simulink model "BLDCMotor"  (R2021a)
settings: Solver=VariableStepAuto  StartTime=0.0  StopTime=1  RelTol=1e-3
undefined symbols (not defined in the file): B, backEMFconstant, J, L, R, torqueConstant
settings Model: Creator=ALAKSHENDRA PC  LastModifiedBy=ALAKSHENDRA PC

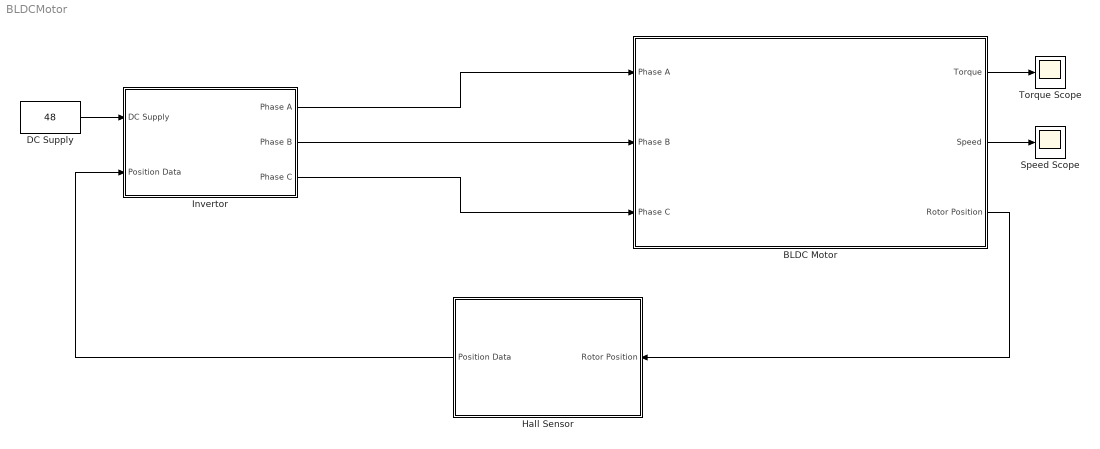
== system BLDCMotor ==
  BLDC Motor : Subsystem
  DC Supply : Constant  Value=48
  Hall Sensor : Subsystem
  Invertor : Subsystem
  Speed Scope : Scope
  Torque Scope : Scope
  wires:
  DC Supply/1 -> Invertor/1(DC Supply)
  Invertor/1(Phase A) -> BLDC Motor/1("Phase A ")
  Invertor/2(Phase B) -> BLDC Motor/2(Phase B)
  Invertor/3(Phase C) -> BLDC Motor/3(Phase C)
  BLDC Motor/3(Rotor Position) -> Hall Sensor/1(Rotor Position)
  Hall Sensor/1(Position Data) -> Invertor/2(Position Data)
  BLDC Motor/1(Torque) -> Torque Scope/1
  BLDC Motor/2(Speed) -> Speed Scope/1

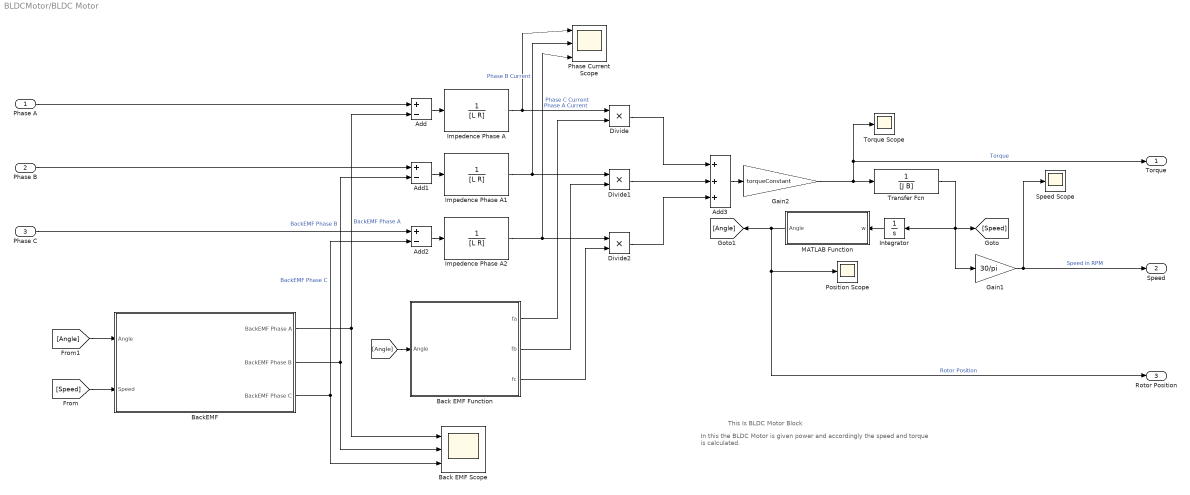
== system BLDCMotor/BLDC Motor ==
  note: This Is BLDC Motor Block
  note: In this the BLDC Motor is given power and accordingly the speed and torque is calculated.
  "Phase A " : Inport
  Phase B : Inport  Port=2
  Phase C : Inport  Port=3
  Add : Sum  Inputs=+-
  Add1 : Sum  Inputs=+-
  Add2 : Sum  Inputs=+-
  Add3 : Sum  Inputs=+++
  Back EMF Function : Subsystem
  Back EMF Scope : Scope  NumInputPorts=3
  BackEMF : Subsystem
  Divide : Product  Inputs=**
  Divide1 : Product  Inputs=**
  Divide2 : Product  Inputs=**
  Gain1 : Gain  Gain=30/pi
  Gain2 : Gain  Gain=torqueConstant
  Impedence Phase A : TransferFcn  Denominator=[L R]
  Impedence Phase A1 : TransferFcn  Denominator=[L R]
  Impedence Phase A2 : TransferFcn  Denominator=[L R]
  Integrator : Integrator
  MATLAB Function : MATLAB Function  TreatAsAtomicUnit=on
  Phase Current Scope : Scope  NumInputPorts=3
  Position Scope : Scope
  Speed Scope : Scope
  Torque Scope : Scope
  Transfer Fcn : TransferFcn  Denominator=[J B]
  Torque : Outport
  Speed : Outport  Port=2
  Rotor Position : Outport  Port=3
  wires:
  Impedence Phase A1/1 -> Divide1/1, Phase Current Scope/2  "Phase B Current"
  [Speed] -> BackEMF/2(Speed)
  BackEMF/2(BackEMF Phase B) -> Back EMF Scope/2, Add1/2  "BackEMF Phase B"
  Add/1 -> Impedence Phase A/1
  Impedence Phase A/1 -> Divide/1, Phase Current Scope/1  "Phase A Current"
  BackEMF/1(BackEMF Phase A) -> Back EMF Scope/1, Add/2  "BackEMF Phase A"
  Back EMF Function/1(fa) -> Divide/2
  BackEMF/3(BackEMF Phase C) -> Back EMF Scope/3, Add2/2  "BackEMF Phase C"
  Back EMF Function/3(fc) -> Divide2/2
  Phase B/1 -> Add1/1
  Add2/1 -> Impedence Phase A2/1
  Integrator/1 -> MATLAB Function/1(w)
  Back EMF Function/2(fb) -> Divide1/2
  Gain2/1 -> Transfer Fcn/1, Torque/1, Torque Scope/1  "Torque"
  Phase C/1 -> Add2/1
  Divide/1 -> Add3/1
  "Phase A "/1 -> Add/1
  MATLAB Function/1(Angle) -> [Angle], Rotor Position/1, Position Scope/1  "Rotor Position"
  Impedence Phase A2/1 -> Divide2/1, Phase Current Scope/3  "Phase C Current"
  Transfer Fcn/1 -> [Speed], Integrator/1, Gain1/1
  Add3/1 -> Gain2/1
  Divide2/1 -> Add3/3
  [Angle] -> Back EMF Function/1(Angle)
  Add1/1 -> Impedence Phase A1/1
  Divide1/1 -> Add3/2
  [Angle] -> BackEMF/1(Angle)
  Gain1/1 -> Speed Scope/1, Speed/1  "Speed in RPM"

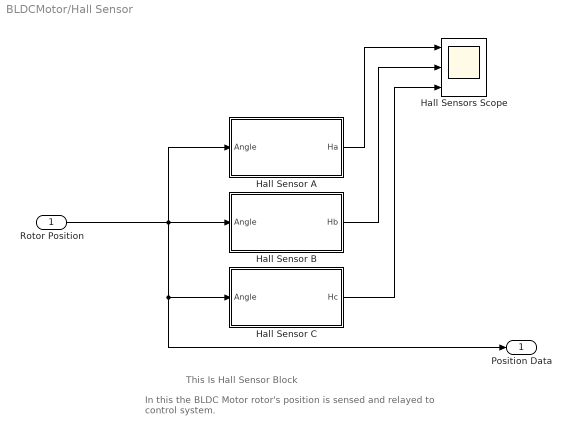
== system BLDCMotor/Hall Sensor ==
  note: This Is Hall Sensor Block
  note: In this the BLDC Motor rotor's position is sensed and relayed to control system.
  Rotor Position : Inport
  Hall Sensor A : MATLAB Function  TreatAsAtomicUnit=on
  Hall Sensor B : MATLAB Function  TreatAsAtomicUnit=on
  Hall Sensor C : MATLAB Function  TreatAsAtomicUnit=on
  Hall Sensors Scope : Scope  NumInputPorts=3
  Position Data : Outport
  wires:
  Hall Sensor B/1(Hb) -> Hall Sensors Scope/2
  Hall Sensor C/1(Hc) -> Hall Sensors Scope/3
  Hall Sensor A/1(Ha) -> Hall Sensors Scope/1
  Rotor Position/1 -> Position Data/1, Hall Sensor C/1(Angle), Hall Sensor A/1(Angle), Hall Sensor B/1(Angle)

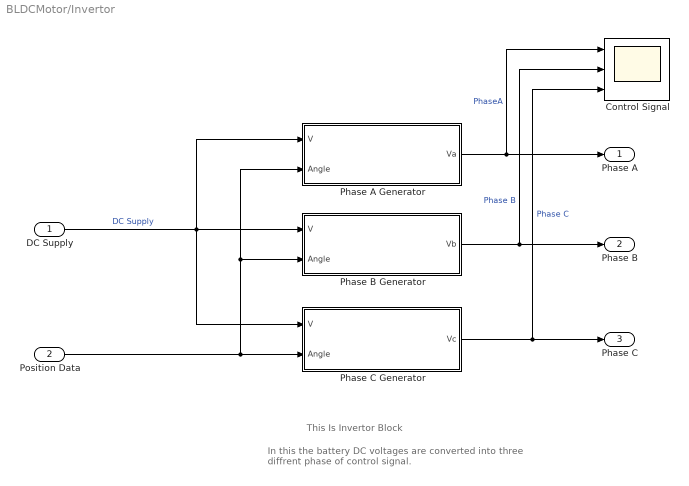
== system BLDCMotor/Invertor ==
  note: In this the battery DC voltages are converted into three diffrent phase of control signal.
  note: This Is Invertor Block
  DC Supply : Inport
  Position Data : Inport  Port=2
  Control Signal : Scope  NumInputPorts=3
  Phase A Generator : MATLAB Function  TreatAsAtomicUnit=on
  Phase B Generator : MATLAB Function  TreatAsAtomicUnit=on
  Phase C Generator : MATLAB Function  TreatAsAtomicUnit=on
  Phase A : Outport
  Phase B : Outport  Port=2
  Phase C : Outport  Port=3
  wires:
  DC Supply/1 -> Phase C Generator/1(V), Phase A Generator/1(V), Phase B Generator/1(V)  "DC Supply"
  Position Data/1 -> Phase A Generator/2(Angle), Phase B Generator/2(Angle), Phase C Generator/2(Angle)
  Phase A Generator/1(Va) -> Control Signal/1, Phase A/1  "PhaseA"
  Phase B Generator/1(Vb) -> Control Signal/2, Phase B/1  "Phase B"
  Phase C Generator/1(Vc) -> Control Signal/3, Phase C/1  "Phase C"

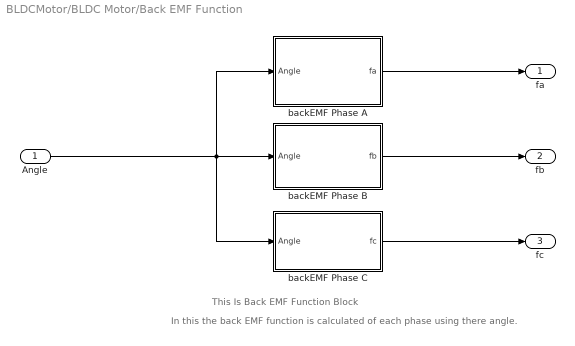
== system BLDCMotor/BLDC Motor/Back EMF Function ==
  note: This Is Back EMF Function Block
  note: In this the back EMF function is calculated of each phase using there angle.
  Angle : Inport
  backEMF Phase A : MATLAB Function  TreatAsAtomicUnit=on
  backEMF Phase B : MATLAB Function  TreatAsAtomicUnit=on
  backEMF Phase C : MATLAB Function  TreatAsAtomicUnit=on
  fa : Outport
  fb : Outport  Port=2
  fc : Outport  Port=3
  wires:
  Angle/1 -> backEMF Phase A/1(Angle), backEMF Phase C/1(Angle), backEMF Phase B/1(Angle)
  backEMF Phase B/1(fb) -> fb/1
  backEMF Phase C/1(fc) -> fc/1
  backEMF Phase A/1(fa) -> fa/1

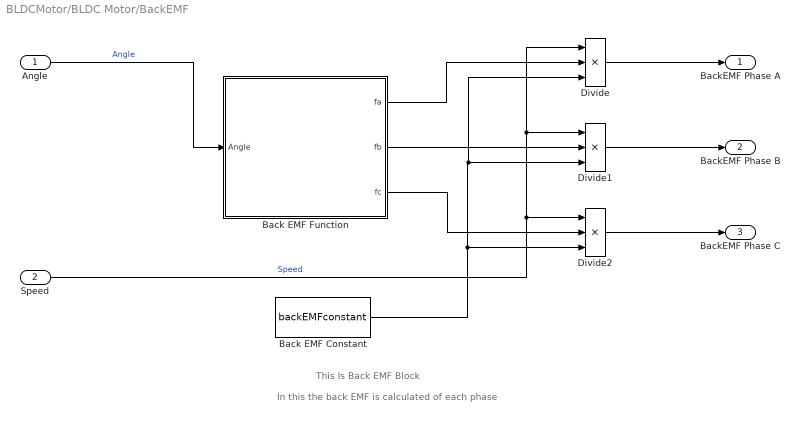
== system BLDCMotor/BLDC Motor/BackEMF ==
  note: This Is Back EMF Block
  note: In this the back EMF is calculated of each phase
  Angle : Inport
  Speed : Inport  Port=2
  Back EMF Constant : Constant  Value=backEMFconstant
  Back EMF Function : Subsystem
  Divide : Product  Inputs=***
  Divide1 : Product  Inputs=***
  Divide2 : Product  Inputs=***
  BackEMF Phase A : Outport
  BackEMF Phase B : Outport  Port=2
  BackEMF Phase C : Outport  Port=3
  wires:
  Back EMF Constant/1 -> Divide/3, Divide1/3, Divide2/3
  Divide1/1 -> BackEMF Phase B/1
  Divide/1 -> BackEMF Phase A/1
  Divide2/1 -> BackEMF Phase C/1
  Speed/1 -> Divide1/1, Divide/1, Divide2/1  "Speed"
  Angle/1 -> Back EMF Function/1(Angle)  "Angle"
  Back EMF Function/1(fa) -> Divide/2
  Back EMF Function/2(fb) -> Divide1/2
  Back EMF Function/3(fc) -> Divide2/2

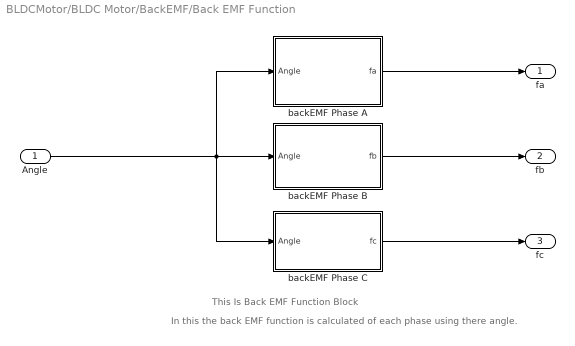
== system BLDCMotor/BLDC Motor/BackEMF/Back EMF Function ==
  note: This Is Back EMF Function Block
  note: In this the back EMF function is calculated of each phase using there angle.
  Angle : Inport
  backEMF Phase A : MATLAB Function  TreatAsAtomicUnit=on
  backEMF Phase B : MATLAB Function  TreatAsAtomicUnit=on
  backEMF Phase C : MATLAB Function  TreatAsAtomicUnit=on
  fa : Outport
  fb : Outport  Port=2
  fc : Outport  Port=3
  wires:
  Angle/1 -> backEMF Phase A/1(Angle), backEMF Phase C/1(Angle), backEMF Phase B/1(Angle)
  backEMF Phase B/1(fb) -> fb/1
  backEMF Phase C/1(fc) -> fc/1
  backEMF Phase A/1(fa) -> fa/1

== matlab function BLDCMotor/Invertor/Phase A Generator ==
  data: V input; Va output; Angle input
function Va = switchLogicPhaseA(V,Angle)
if Angle<=pi/3 && Angle >= 0
    Va = V;
elseif Angle>=pi/3 && Angle <= pi*2/3
    Va = V;
elseif Angle>=pi*2/3 && Angle <= pi
    Va = 0;
elseif Angle>=pi && Angle <= pi*4/3
    Va = -V;
elseif Angle>=pi*4/3 && Angle <= pi*5/3
    Va = -V;
else
    Va = 0;
end
end

== matlab function BLDCMotor/Invertor/Phase C Generator ==
  data: V input; Vc output; Angle input
function Vc = switchLogicPhaseC(V,Angle)
if Angle<=pi/3 && Angle >= 0
    Vc = 0;
elseif Angle>=pi/3 && Angle <= pi*2/3
    Vc = -V;
elseif Angle>=pi*2/3 && Angle <= pi
    Vc = -V;
elseif Angle>=pi && Angle <= pi*4/3
    Vc = 0;
elseif Angle>=pi*4/3 && Angle <= pi*5/3
    Vc = V;
else
    Vc = V;
end
end

== matlab function BLDCMotor/Hall Sensor/Hall Sensor A ==
  data: Angle input; Ha output
function Ha = hallSensorA(Angle)
if Angle<=pi/3 && Angle >= 0
    Ha = 1;
elseif Angle>=pi/3 && Angle <= pi*2/3
    Ha = 1;
elseif Angle>=pi*2/3 && Angle <= pi
    Ha = 0;
elseif Angle>=pi && Angle <= pi*4/3
    Ha = 0;
elseif Angle>=pi*4/3 && Angle <= pi*5/3
    Ha = 0;
else
    Ha = 1;
end
end

== matlab function BLDCMotor/Hall Sensor/Hall Sensor B ==
  data: Angle input; Hb output
function Hb = hallSensorB(Angle)
if Angle<=pi/3 && Angle >= 0
    Hb = 0;
elseif Angle>=pi/3 && Angle <= pi*2/3
    Hb = 1;
elseif Angle>=pi*2/3 && Angle <= pi
    Hb = 1;
elseif Angle>=pi && Angle <= pi*4/3
    Hb = 1;
elseif Angle>=pi*4/3 && Angle <= pi*5/3
    Hb = 0;
else
    Hb = 0;
end
end

== matlab function BLDCMotor/Hall Sensor/Hall Sensor C ==
  data: Angle input; Hc output
function Hc = hallSensorC(Angle)
if Angle<=pi/3 && Angle >= 0
    Hc = 0;
elseif Angle>=pi/3 && Angle <= pi*2/3
    Hc = 0;
elseif Angle>=pi*2/3 && Angle <= pi
    Hc = 0;
elseif Angle>=pi && Angle <= pi*4/3
    Hc = 1;
elseif Angle>=pi*4/3 && Angle <= pi*5/3
    Hc = 1;
else
    Hc = 1;
end
end

== matlab function BLDCMotor/BLDC Motor/BackEMF/Back EMF Function/backEMF Phase A ==
  data: Angle input; fa output
function fa = backEMFa(Angle)
    if Angle >= 0 && Angle <= pi/6
        fa = 6*Angle/pi;
    elseif Angle >= pi/6 && Angle <= pi*5/6
        fa = 1;
    elseif Angle >= pi*5/6 && Angle <= pi*7/6
        fa = -6*Angle/pi + 6;
    elseif Angle >= pi*7/6 && Angle <= pi*11/6
        fa = -1;
    else 
        fa = 6*Angle/pi - 12;
    end
end

== matlab function BLDCMotor/BLDC Motor/BackEMF/Back EMF Function/backEMF Phase B ==
  data: Angle input; fb output
function fb = backEMFb(Angle)
    if Angle >= 0 && Angle <= pi/2
        fb = -1;
    elseif Angle >= pi/2 && Angle <= pi*5/6
        fb = 6*Angle/pi - 4;
    elseif Angle >= pi*5/6 && Angle <= pi*9/6
        fb = 1;
    elseif Angle >= pi*9/6 && Angle <= pi*11/6
        fb = -6*Angle/pi + 10;
    else 
        fb = -1;
    end
end

== matlab function BLDCMotor/BLDC Motor/BackEMF/Back EMF Function/backEMF Phase C ==
  data: Angle input; fc output
function fc = backEMFc(Angle)
    if Angle >= 0 && Angle <= pi/6
        fc = 1;
    elseif Angle >= pi/6 && Angle <= pi/2
        fc = -6*Angle/pi + 2;
    elseif Angle >= pi/2 && Angle <= pi*7/6
        fc = -1;
    elseif Angle >= pi*7/6 && Angle <= pi*9/6
        fc = 6*Angle/pi - 8;
    else 
        fc = 1;
    end
end

== matlab function BLDCMotor/BLDC Motor/Back EMF Function/backEMF Phase A ==
  data: Angle input; fa output
function fa = backEMFa(Angle)
    if Angle >= 0 && Angle <= pi/6
        fa = 6*Angle/pi;
    elseif Angle >= pi/6 && Angle <= pi*5/6
        fa = 1;
    elseif Angle >= pi*5/6 && Angle <= pi*7/6
        fa = -6*Angle/pi + 6;
    elseif Angle >= pi*7/6 && Angle <= pi*11/6
        fa = -1;
    else 
        fa = 6*Angle/pi - 12;
    end
end

== matlab function BLDCMotor/Invertor/Phase B Generator ==
  data: V input; Vb output; Angle input
function Vb = switchLogicPhaseB(V,Angle)
if Angle<=pi/3 && Angle >= 0
    Vb = -V;
elseif Angle>=pi/3 && Angle <= pi*2/3
    Vb = 0;
elseif Angle>=pi*2/3 && Angle <= pi
    Vb = V;
elseif Angle>=pi && Angle <= pi*4/3
    Vb = V;
elseif Angle>=pi*4/3 && Angle <= pi*5/3
    Vb = 0;
else
    Vb = -V;
end
end

== matlab function BLDCMotor/BLDC Motor/Back EMF Function/backEMF Phase B ==
  data: Angle input; fb output
function fb = backEMFb(Angle)
    if Angle >= 0 && Angle <= pi/2
        fb = -1;
    elseif Angle >= pi/2 && Angle <= pi*5/6
        fb = 6*Angle/pi - 4;
    elseif Angle >= pi*5/6 && Angle <= pi*9/6
        fb = 1;
    elseif Angle >= pi*9/6 && Angle <= pi*11/6
        fb = -6*Angle/pi + 10;
    else 
        fb = -1;
    end
end

== matlab function BLDCMotor/BLDC Motor/Back EMF Function/backEMF Phase C ==
  data: Angle input; fc output
function fc = backEMFc(Angle)
    if Angle >= 0 && Angle <= pi/6
        fc = 1;
    elseif Angle >= pi/6 && Angle <= pi/2
        fc = -6*Angle/pi + 2;
    elseif Angle >= pi/2 && Angle <= pi*7/6
        fc = -1;
    elseif Angle >= pi*7/6 && Angle <= pi*9/6
        fc = 6*Angle/pi - 8;
    else 
        fc = 1;
    end
end

== matlab function BLDCMotor/BLDC Motor/MATLAB Function ==
  data: w input; Angle output
function Angle = angleCorrection(w)
    Angle = mod(w,2*pi);
end
